simulink model "MDS_PID"  (R2015a)
settings: Solver=ode45  StartTime=0.0  StopTime=100  RelTol=1e-3  AbsTol=1e-6
libraries: cstblocks x4
settings Model: Creator=ANILKUMAR  LastModifiedBy=ANILKUMAR

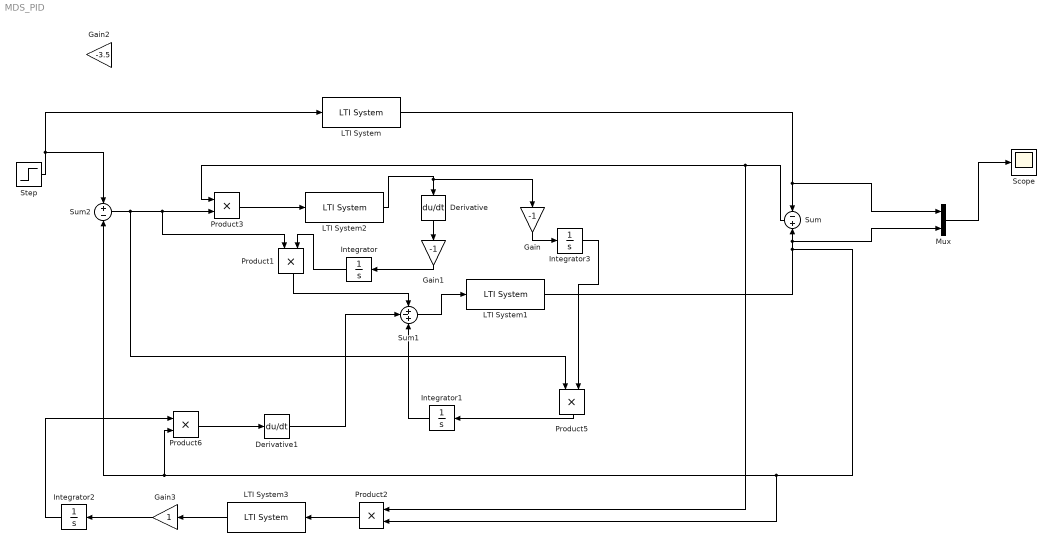
== system MDS_PID ==
  Derivative : Derivative
  Derivative1 : Derivative
  Gain : Gain  Gain=-1
  Gain1 : Gain  Gain=-1
  Gain2 : Gain  Gain=-3.5
  Gain3 : Gain
  Integrator{,1..3} (4 alike) : Integrator
  LTI System : cstblocks/LTI System  sys=tf(25,[1 6 25])  IC=[]
  LTI System1 : cstblocks/LTI System  sys=tf(.3,[1 .3 .6])  IC=[]
  LTI System2 : cstblocks/LTI System  sys=tf(1,[1 6 25])  IC=[]
  LTI System3 : cstblocks/LTI System  sys=tf([1,0,0],[1 6 25])  IC=[]
  Mux : Mux  Inputs=2
  Product{1..3,5..6} (5 alike) : Product
  Scope : Scope
      settings: YMin=0  YMax=575
  Step : Step  Time=0  SampleTime=0
  Sum : Sum  Inputs=-+
  Sum1 : Sum  Inputs=+-+
  Sum2 : Sum  Inputs=+-
  wires:
  LTI System/1 -> Mux/1, Sum/1
  LTI System1/1 -> Product2/2, Product6/2, Sum2/2, Mux/2, Sum/2
  Step/1 -> Sum2/1, LTI System/1
  Sum2/1 -> Product5/1, Product1/1, Product3/2
  Sum/1 -> Product2/1, Product3/1
  Product3/1 -> LTI System2/1
  LTI System2/1 -> Gain/1, Derivative/1
  Derivative/1 -> Gain1/1
  Gain1/1 -> Integrator/1
  Integrator/1 -> Product1/2
  Sum1/1 -> LTI System1/1
  Product1/1 -> Sum1/1
  Gain/1 -> Integrator3/1
  Integrator3/1 -> Product5/2
  Product5/1 -> Integrator1/1
  Integrator1/1 -> Sum1/3
  Product2/1 -> LTI System3/1
  LTI System3/1 -> Gain3/1
  Product6/1 -> Derivative1/1
  Derivative1/1 -> Sum1/2
  Mux/1 -> Scope/1
  Gain3/1 -> Integrator2/1
  Integrator2/1 -> Product6/1
